simulink model "kcm_cosim"  (Simulink 6.4)
settings: Solver=FixedStepDiscrete  SolverMode=SingleTasking  StartTime=0.0  StopTime=1e-1  RelTol=1e-3
undefined symbols (not defined in the file or in its folder): pipeline_prec
libraries: modelsimlib x5
settings Model: LastModifiedBy=Administrador

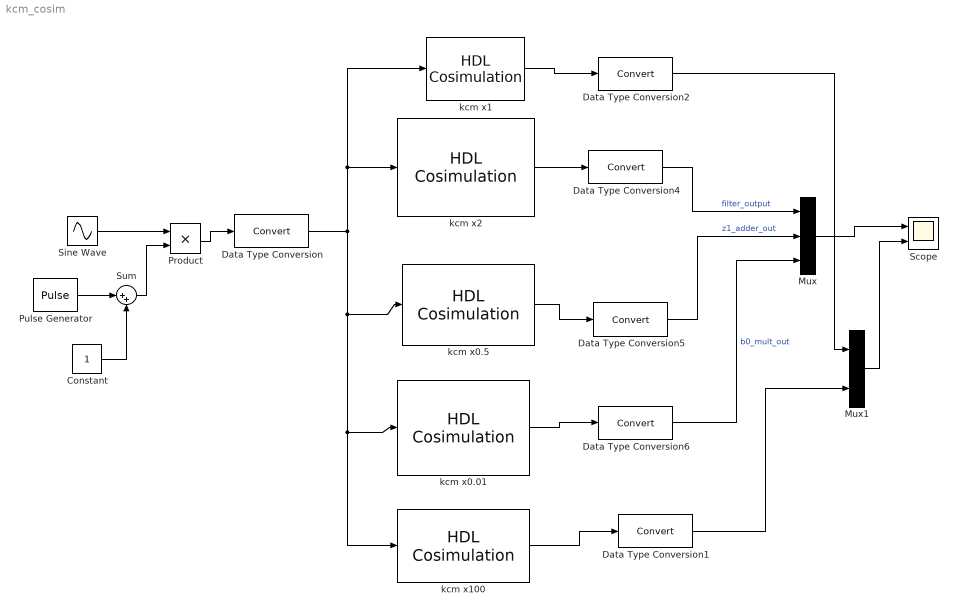
== system kcm_cosim ==
  Constant : Constant  Value=1  OutDataType=sfix(16)  ConRadixGroup=Use specified scaling  OutScaling=2^0  SampleTime=inf  FramePeriod=inf
  Data Type Conversion : DataTypeConversion  OutDataTypeMode=Specify via dialog  OutScaling=2^(-pipeline_prec)  RndMeth=Nearest  SampleTime=1e-4  SaturateOnIntegerOverflow=on
  Data Type Conversion{1..2,4..6} (5 alike) : DataTypeConversion  OutDataTypeMode=double
  Mux : Mux  Inputs=3
  Mux1 : Mux  Inputs=2
  Product : Product  RndMeth=Zero
  Pulse Generator : DiscretePulseGenerator  PulseType=Time based  Amplitude=4  Period=2/50  PulseWidth=50
  Scope : Scope  NumInputPorts=2
      settings: TimeRange=0.01  YMin=-1~-5  YMax=1~5  MaxDataPoints=500000
  Sine Wave : Sin  Frequency=2*pi*50
  Sum : Sum  Inputs=|++
  kcm x0.01 : modelsimlib/HDL Cosimulation  DialogController=modelsimddg.CoSim  DialogControllerArgs=DataTag0  PortPaths=/kcm_cosim_tb/kcm_001_i/i;/kcm_cosim_tb/kcm_001_i/o  PortModes=[1 2 ]  PortTimes=[1,1e-4]  PortSigns=[-1 1 ]  PortFracLengths=[0,pipeline_prec]  CommLocal=on  CommSharedMemory=off  CommPortNumber=4449  CommShowInfo=on  ClockModes=[]  ClockTimes=[]  TclPreSimCommand="echo \"Running Simulink Cosimulation block.\""  TclPostSimCommand="echo \"done\""  TimingMode=s  TimingScaleFactor=1  idxCellArray={'UNUSED_VAR'}
  kcm x0.5 : modelsimlib/HDL Cosimulation  DialogController=modelsimddg.CoSim  DialogControllerArgs=DataTag1  PortPaths=/kcm_cosim_tb/kcm_05_i/i;/kcm_cosim_tb/kcm_05_i/o  PortModes=[1 2 ]  PortTimes=[1,1e-4]  PortSigns=[-1 1 ]  PortFracLengths=[0,pipeline_prec]  CommLocal=on  CommSharedMemory=off  CommPortNumber=4449  CommShowInfo=on  ClockModes=[]  ClockTimes=[]  TclPreSimCommand="echo \"Running Simulink Cosimulation block.\""  TclPostSimCommand="echo \"done\""  TimingMode=s  TimingScaleFactor=1  idxCellArray={'UNUSED_VAR'}
  kcm x1 : modelsimlib/HDL Cosimulation  DialogController=modelsimddg.CoSim  DialogControllerArgs=DataTag2  PortPaths=/kcm_cosim_tb/kcm_m233_i/i;/kcm_cosim_tb/kcm_m233_i/o  PortModes=[1 2 ]  PortTimes=[1,1e-4]  PortSigns=[-1 1 ]  PortFracLengths=[0,pipeline_prec]  CommLocal=on  CommSharedMemory=off  CommPortNumber=4449  CommShowInfo=on  ClockModes=[]  ClockTimes=[]  TclPreSimCommand="echo \"Running Simulink Cosimulation block.\""  TclPostSimCommand="echo \"done\""  TimingMode=s  TimingScaleFactor=1  idxCellArray={'UNUSED_VAR'}
  kcm x100 : modelsimlib/HDL Cosimulation  DialogController=modelsimddg.CoSim  DialogControllerArgs=DataTag3  PortPaths=/kcm_cosim_tb/kcm_100_i/i;/kcm_cosim_tb/kcm_100_i/o  PortModes=[1 2 ]  PortTimes=[1,1e-4]  PortSigns=[-1 1 ]  PortFracLengths=[0,pipeline_prec]  CommLocal=on  CommSharedMemory=off  CommPortNumber=4449  CommShowInfo=on  ClockModes=[]  ClockTimes=[]  TclPreSimCommand="echo \"Running Simulink Cosimulation block.\""  TclPostSimCommand="echo \"done\""  TimingMode=s  TimingScaleFactor=1  idxCellArray={'UNUSED_VAR'}
  kcm x2 : modelsimlib/HDL Cosimulation  DialogController=modelsimddg.CoSim  DialogControllerArgs=DataTag4  PortPaths=/kcm_cosim_tb/kcm_2_i/i;/kcm_cosim_tb/kcm_2_i/o  PortModes=[1 2 ]  PortTimes=[1,1e-4]  PortSigns=[-1 1 ]  PortFracLengths=[0,pipeline_prec]  CommLocal=on  CommSharedMemory=off  CommPortNumber=4449  CommShowInfo=on  ClockModes=[]  ClockTimes=[]  TclPreSimCommand="echo \"Running Simulink Cosimulation block.\""  TclPostSimCommand="echo \"done\""  TimingMode=s  TimingScaleFactor=1  idxCellArray={'UNUSED_VAR'}
  wires:
  Data Type Conversion/1 -> kcm x0.5/1, kcm x0.01/1, kcm x100/1, kcm x2/1, kcm x1/1
  kcm x2/1 -> Data Type Conversion4/1
  kcm x0.5/1 -> Data Type Conversion5/1
  kcm x0.01/1 -> Data Type Conversion6/1
  kcm x100/1 -> Data Type Conversion1/1
  Data Type Conversion4/1 -> Mux/1  "filter_output"
  Data Type Conversion5/1 -> Mux/2  "z1_adder_out"
  Data Type Conversion6/1 -> Mux/3  "b0_mult_out"
  Mux/1 -> Scope/1
  Pulse Generator/1 -> Sum/1
  Constant/1 -> Sum/2
  Sine Wave/1 -> Product/1
  Product/1 -> Data Type Conversion/1
  Sum/1 -> Product/2
  Mux1/1 -> Scope/2
  Data Type Conversion1/1 -> Mux1/2
  kcm x1/1 -> Data Type Conversion2/1
  Data Type Conversion2/1 -> Mux1/1
